simulink model "ExercicioAvaliativo_4"  (R2018a)
settings: Solver=VariableStepAuto  StartTime=0.0  StopTime=10.0  RelTol=1e-3
settings Model: Creator=Particular  LastModifiedBy=Particular

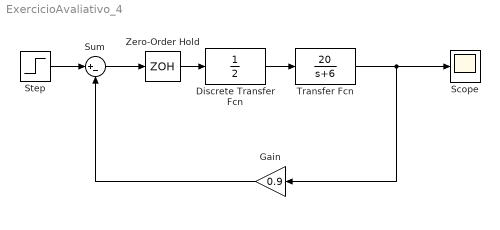
== system ExercicioAvaliativo_4 ==
  Discrete Transfer Fcn : DiscreteTransferFcn  Denominator=[2]
  Gain : Gain  Gain=0.9
  Scope : Scope
  Step : Step  SampleTime=0
  Sum : Sum  Inputs=|+-
  Transfer Fcn : TransferFcn  Numerator=[20]  Denominator=[1 6]
  Zero-Order Hold : ZeroOrderHold  SampleTime=0.05
  wires:
  Transfer Fcn/1 -> Gain/1, Scope/1
  Gain/1 -> Sum/2
  Sum/1 -> Zero-Order Hold/1
  Zero-Order Hold/1 -> Discrete Transfer Fcn/1
  Discrete Transfer Fcn/1 -> Transfer Fcn/1
  Step/1 -> Sum/1
